simulink model "DirectKinematics_Test"  (R2023b)
settings: Solver=VariableStepAuto  StartTime=0.0  StopTime=10.0  RelTol=1e-3
undefined symbols (not defined in the file or in its folder): a, b
settings Model: Creator=eliasoa  LastModifiedBy=eliasoa

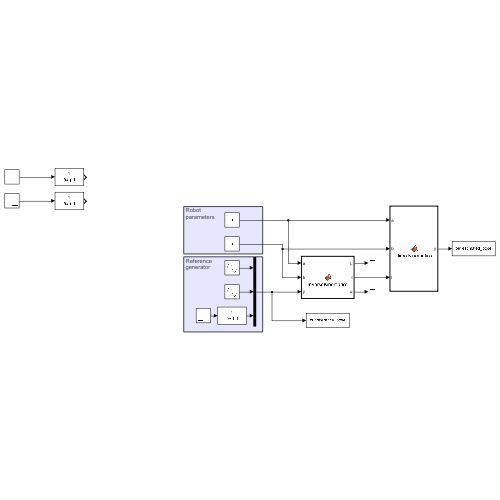
[thumbnail: Simulink's stored preview of the top-level diagram]
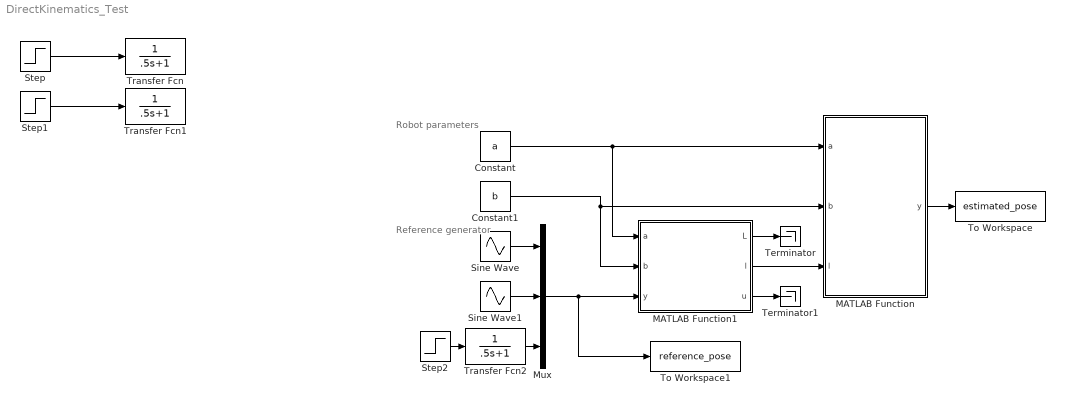
== system DirectKinematics_Test ==
  note: Robot
      | parameters
  note: Reference
      | generator
  Constant : Constant  Value=a
  Constant1 : Constant  Value=b
  MATLAB Function : MATLAB Function  TreatAsAtomicUnit=on
  MATLAB Function1 : MATLAB Function  TreatAsAtomicUnit=on
  Mux : Mux  Inputs=3
  Sine Wave : Sin  Amplitude=.3  SampleTime=0
  Sine Wave1 : Sin  Amplitude=.3  Phase=pi/2  SampleTime=0
  Step : Step  After=0.4  SampleTime=0
  Step1 : Step  After=-0.3  SampleTime=0
  Step2 : Step  After=30*pi/180  SampleTime=0
  Terminator : Terminator
  Terminator1 : Terminator
  To Workspace : ToWorkspace  VariableName=estimated_pose  SaveFormat=Structure With Time  SampleTime=-1
  To Workspace1 : ToWorkspace  VariableName=reference_pose  SaveFormat=Structure With Time  SampleTime=-1
  Transfer Fcn : TransferFcn  Denominator=[.5 1]
  Transfer Fcn1 : TransferFcn  Denominator=[.5 1]
  Transfer Fcn2 : TransferFcn  Denominator=[.5 1]
  wires:
  Constant/1 -> MATLAB Function1/1(a), MATLAB Function/1(a)
  Constant1/1 -> MATLAB Function1/2(b), MATLAB Function/2(b)
  MATLAB Function1/2(l) -> MATLAB Function/3(l)
  MATLAB Function1/1(L) -> Terminator/1
  MATLAB Function1/3(u) -> Terminator1/1
  Step2/1 -> Transfer Fcn2/1
  Step/1 -> Transfer Fcn/1
  Step1/1 -> Transfer Fcn1/1
  Transfer Fcn2/1 -> Mux/3
  Mux/1 -> To Workspace1/1, MATLAB Function1/3(y)
  MATLAB Function/1(y) -> To Workspace/1
  Sine Wave/1 -> Mux/1
  Sine Wave1/1 -> Mux/2

== matlab function DirectKinematics_Test/MATLAB Function1 ==
  data: a input; L output; b input; y input; l output; u output
function [L,l,u] = InverseKinematics(a, b, y)
[L,l,u] = InverseKinematics(a, b, y);
end

== matlab function DirectKinematics_Test/MATLAB Function ==
  data: a input; y output; b input; l input
function y  = DirectKinematics(a,b,l)
    [y] = DirectKinematics(a,b,l);
end
